simulink model "chap10_3sim"  (Simulink 7.7)
settings: Solver=FixedStepDiscrete  StartTime=0.0  StopTime=2  RelTol=1e-3
values from neighbouring files (symbols this model uses):
  A = [1 0.0010 ... (first row only)    [chap10_1.m]    (also in chap10_3ctrl.m = [1.0000    0.0010; chap10_7.m = A1; chap10_8.m = A1)
  B = [-0.0001 ... (first row only)    [chap10_1.m]    (also in chap10_3ctrl.m = [0.0001; chap10_7.m = [0;b]; chap10_8.m = B1)
  C = [c 1]    [chap10_1.m]    (also in chap10_7.m = [1,0]; chap10_8.m = [c,1])
  D = 0    [chap10_7.m]
  T = 0.001    [chap10_3ctrl.m]    (also in chap10_3int.m)
settings Model: Creator=ljk  LastModifiedBy=ljk  ExtModeTrigMode=oneshot  ExtModeArmWhenConnect=off
settings DataIOCC: Decimation=100  LimitDataPoints=off  SaveOutput=off  SaveTime=off
settings OptimizationCC: BlockReduction=off  BooleanDataType=off
settings DebuggingCC: SaveWithParameterizedLinksMsg=none  SignalResolutionControl=TryResolveAllWithWarning  SolverPrmCheckMsg=none  MultiTaskDSMMsg=warning  MultiTaskCondExecSysMsg=none  StrictBusMsg=None
settings HardwareCC: TargetUnknown=on
settings RTWCC: IncludeERTFirstTime=on

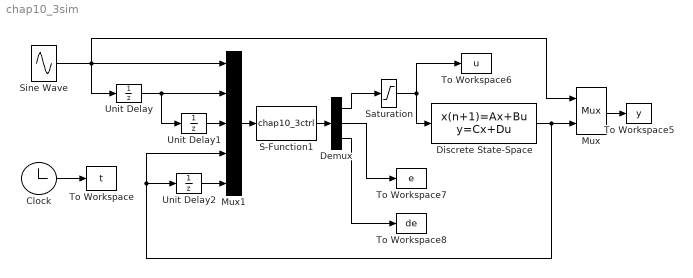
== system chap10_3sim ==
  Clock : Clock
  Demux : Demux  Outputs=3
  Discrete State-Space : DiscreteStateSpace  A=A  B=B  C=C  D=D  X0=[-0.5,-0.5]  SampleTime=T
  Mux : Mux  Inputs=2
  Mux1 : Mux  Inputs=5
  S-Function1 : S-Function  FunctionName=chap10_3ctrl  EnableBusSupport=off
  Saturation : Saturate  UpperLimit=10  LowerLimit=-10
  Sine Wave : Sin  Amplitude=0.5  Frequency=3*2*pi  SampleTime=0.001
  To Workspace : ToWorkspace  VariableName=t  SampleTime=-1  SaveFormat=Array
  To Workspace5 : ToWorkspace  VariableName=y  SampleTime=-1  SaveFormat=Array
  To Workspace6 : ToWorkspace  VariableName=u  SampleTime=-1  SaveFormat=Array
  To Workspace7 : ToWorkspace  VariableName=e  SampleTime=-1  SaveFormat=Array
  To Workspace8 : ToWorkspace  VariableName=de  SampleTime=-1  SaveFormat=Array
  Unit Delay : UnitDelay  SampleTime=0.001
  Unit Delay1 : UnitDelay  SampleTime=0.001
  Unit Delay2 : UnitDelay  SampleTime=0.001
  wires:
  Mux/1 -> To Workspace5/1
  Mux1/1 -> S-Function1/1
  Discrete State-Space/1 -> Mux/2, Mux1/4, Unit Delay2/1
  Sine Wave/1 -> Mux/1, Unit Delay/1, Mux1/1
  Unit Delay1/1 -> Mux1/3
  Unit Delay/1 -> Mux1/2, Unit Delay1/1
  Unit Delay2/1 -> Mux1/5
  Clock/1 -> To Workspace/1
  S-Function1/1 -> Demux/1
  Demux/2 -> To Workspace7/1
  Demux/3 -> To Workspace8/1
  Demux/1 -> Saturation/1
  Saturation/1 -> Discrete State-Space/1, To Workspace6/1
